simulink model "flightcode"  (Simulink 7.5)
settings: Solver=FixedStepDiscrete  StartTime=0.0  StopTime=10.0  FixedStep=SampleTime  RelTol=1e-3
libraries: simulink x1
settings Model: Creator=austinmurch  LastModifiedBy=austinmurch
settings OptimizationCC: InlineParams=on  SimCompilerOptimization=On
settings DebuggingCC: StrictBusMsg=Warning
settings HardwareCC: ProdIntDivRoundTo=Zero  ProdEndianess=BigEndian  ProdHWDeviceType=Freescale->32-bit PowerPC
settings ModelReferenceCC: ModelReferenceNumInstancesAllowed=Single

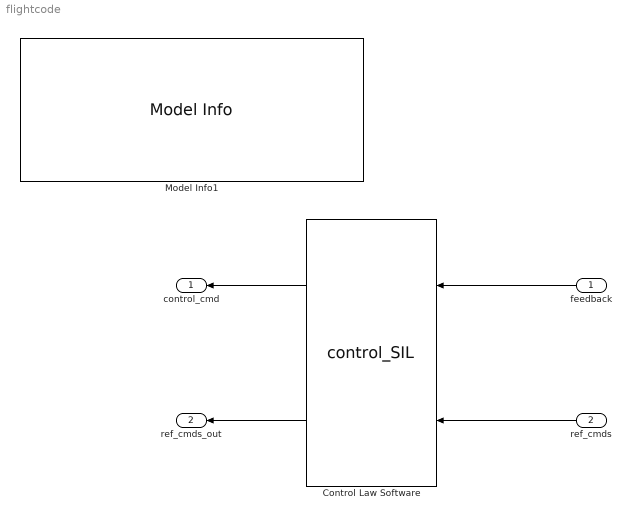
== system flightcode ==
  feedback : Inport
  ref_cmds : Inport  Port=2
  Control Law Software : S-Function  FunctionName=control_SIL  Parameters=SampleTime  EnableBusSupport=off
  Model Info1 : simulink/Model-Wide Utilities/Model Info  SystemSampleTime=-1  InitialBlockCM=None  BlockCM=None  Frame=on  DisplayStringWithTags=|  HorizontalTextAlignment=Left  LeftAlignmentValue=0.02  SourceBlockDiagram=flightcode  TagMaxNumber=20
      | MODEL INFORMATION
      | Flight code implementation of controller code in C
      | 
      | University of Minnesota
      | Aerospace Engineering and Mechanics
      | Copyright 2011 Regents of the University of Minnesota. All rights reserved.
      | 
      | == SVN Info ==
      | %<ModelVersion>
      | Last modified by %<LastModifiedBy> on %<LastModificationDate>
  control_cmd : Outport
  ref_cmds_out : Outport  Port=2
  wires:
  feedback/1 -> Control Law Software/1
  ref_cmds/1 -> Control Law Software/2
  Control Law Software/1 -> control_cmd/1
  Control Law Software/2 -> ref_cmds_out/1
